simulink model "modello_la_disturbo"  (R2023a)
settings: Solver=VariableStepAuto  StartTime=0.0  StopTime=10.0  RelTol=1e-3
values from neighbouring files (symbols this model uses):
  K_sim = K_H2_HINF    [LA.m]
  parametri = [V_1, L, d, alpha, beta]    [LA.m]
  x_0 = [0; 0; 0]    [LA.m]
  x_eq = [0; 0; 0]    [LA.m]
undefined symbols (not defined in the file or in its folder): sigbuilder_block
libraries: simulink x1
settings Model: Creator=Randy  LastModifiedBy=Randy

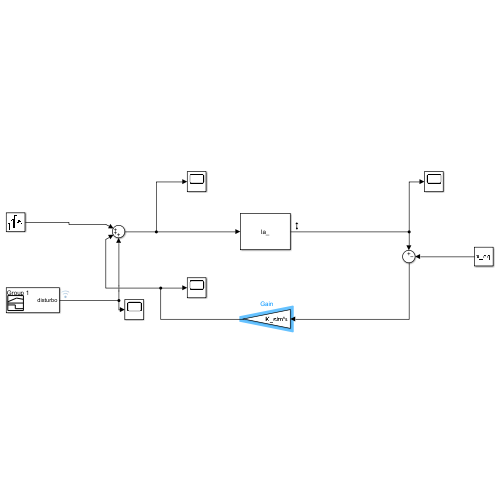
[thumbnail: Simulink's stored preview of the top-level diagram]
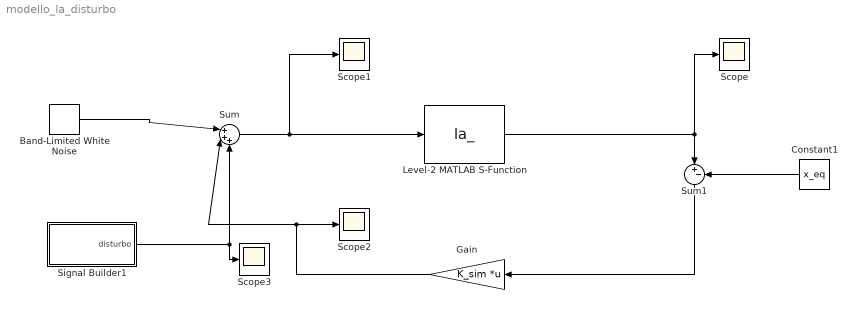
== system modello_la_disturbo ==
  Band-Limited White Noise : simulink/Sources/Band-Limited White Noise  Cov=[0.01]  Ts=0.1  seed=[23341]
  Constant1 : Constant  Value=x_eq
  Gain : Gain  Gain=K_sim  Multiplication=Matrix(K*u)
  Level-2 MATLAB S-Function : M-S-Function  FunctionName=la_  Parameters=x_0,parametri
  Scope{,1..3} (4 alike) : Scope
  Signal Builder1 : Subsystem  Tag=STV Subsys  LoadFcn=sigbuilder_block('load');  StartFcn=sigbuilder_block('start');  StopFcn=sigbuilder_block('stop');  ClipboardFcn=sigbuilder_block('clipboard');  mask(Sigbuilder block){tuvar=[0:10]}
      mask help: Simulink:masks:SigbuilderBlock_MD
      mask init:
      | if ~strcmp(get_param(bdroot(gcbh),'SimulationStatus'),'stopped') tuvar = sigbuilder_block('maskInit'); end
      settings: CopyFcn=sigbuilder_block('copy');  DeleteFcn=sigbuilder_block('delete');  ModelCloseFcn=sigbuilder_block('modelClose');  PreSaveFcn=sigbuilder_block('preSave');  PauseFcn=sigbuilder_block('pause');  ContinueFcn=sigbuilder_block('continue');  NameChangeFcn=sigbuilder_block('namechange');  OpenFcn=sigbuilder_block('open',[6 30 1012.5 470.25 ]);  CloseFcn=sigbuilder_block('close');
      mask Display: plot(0, 0, 100, 100,[2, 2, 32, 32, 2], [68, 8, 8, 68, 68],[32, 2], [38, 38], [32, 19, 2],[53, 60, 44], [32, 17, 17, 2],[16, 16, 31, 31]);txt = getActiveGroup(gcbh);text(2, 100, txt,'verticalAlignment', 'top');
  Sum : Sum  Inputs=|+++
  Sum1 : Sum  Inputs=|+-
  wires:
  Signal Builder1/1(disturbo) -> Sum/3, Scope3/1
  Sum/1 -> Scope1/1, Level-2 MATLAB S-Function/1
  Level-2 MATLAB S-Function/1 -> Scope/1, Sum1/1
  Sum1/1 -> Gain/1
  Gain/1 -> Scope2/1, Sum/2
  Constant1/1 -> Sum1/2
  Band-Limited White Noise/1 -> Sum/1

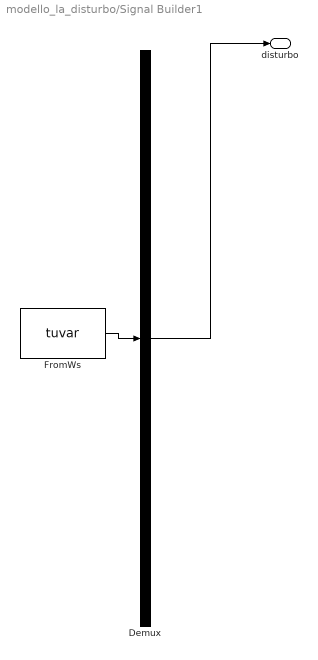
== system modello_la_disturbo/Signal Builder1 ==
  Demux : Demux  Tag=STV Demux  Outputs=1
      settings: DisplayOption=none
  FromWs : FromWorkspace  Tag=STV FromWs  VariableName=tuvar
      SigBuilderData=|
      | common.afterFinalStr = 'Extrapolate'
      | common.sampleTime = 0
      | dataSet.timeRange = [0 20]
      | dataSet.name = 'Group 1'
      | sbobj.Groups.Name = 'Group 1'
      | sbobj.Groups.Signals.Name = 'disturbo'
      | sbobj.Groups.Signals.XData = [0 2 2 4 4 15 20]
      | sbobj.Groups.Signals.YData = [0 0 2 2 0 0 0]
      | sbobj.Groups.TimeRange = [0 20]
  disturbo : Outport  Tag=STV Outport  VectorParamsAs1DForOutWhenUnconnected=off
  wires:
  Demux/1 -> disturbo/1
  FromWs/1 -> Demux/1
